simulink model "SUPERSONIC_SIMULINK"  (R2020a)
settings: Solver=VariableStepAuto  StartTime=0.0  StopTime=2.5  RelTol=1e-3
values from neighbouring files (symbols this model uses):
  K = 0.815    [SUPERSONIC_SAS.m]
libraries: cstblocks x1
settings Model: Creator=AHSAN  LastModifiedBy=AHSAN

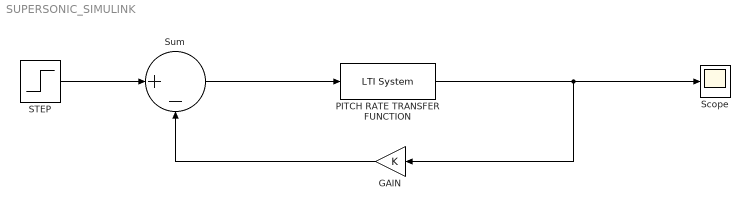
== system SUPERSONIC_SIMULINK ==
  "GAIN " : Gain  Gain=K
  PITCH RATE TRANSFER FUNCTION : cstblocks/LTI System  sys=PitchRate_TF  IC=[]
  STEP : Step  Time=0  SampleTime=0
  Scope : Scope
  Sum : Sum  Inputs=|+-
  wires:
  Sum/1 -> PITCH RATE TRANSFER FUNCTION/1
  PITCH RATE TRANSFER FUNCTION/1 -> "GAIN "/1, Scope/1
  "GAIN "/1 -> Sum/2
  STEP/1 -> Sum/1
